simulink model "Task_2a"  (R2021b)
settings: Solver=VariableStepAuto  StartTime=0.0  StopTime=100.0  FixedStep=0.01`  RelTol=1e-3
model workspace (MAT data in the model file):
  Kd = 1
  Ki = 22
  Kp = 200
  Ts = 0.01
  b = 50
  m = 1000
  u = 500
settings Model: Creator=mluser  LastModifiedBy=mluser

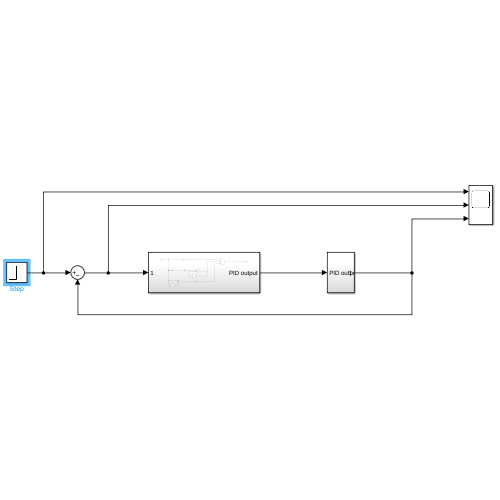
[thumbnail: Simulink's stored preview of the top-level diagram]
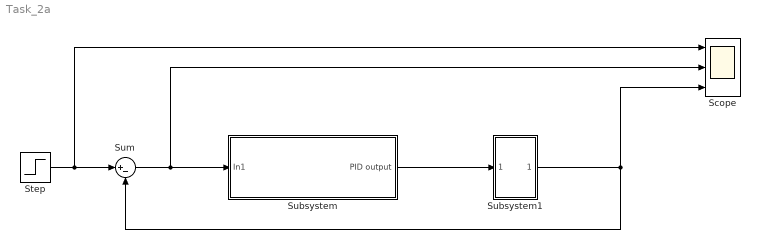
== system Task_2a ==
  Scope : Scope  NumInputPorts=3
  Step : Step  Time=0  After=u  SampleTime=0.01
  Subsystem : Subsystem
  Subsystem1 : Subsystem
  Sum : Sum  Inputs=|+-
  wires:
  Step/1 -> Sum/1, Scope/1
  Subsystem1/1(Out1) -> Sum/2, Scope/3
  Sum/1 -> Subsystem/1(In1), Scope/2
  Subsystem/1(PID output) -> Subsystem1/1(PID output)

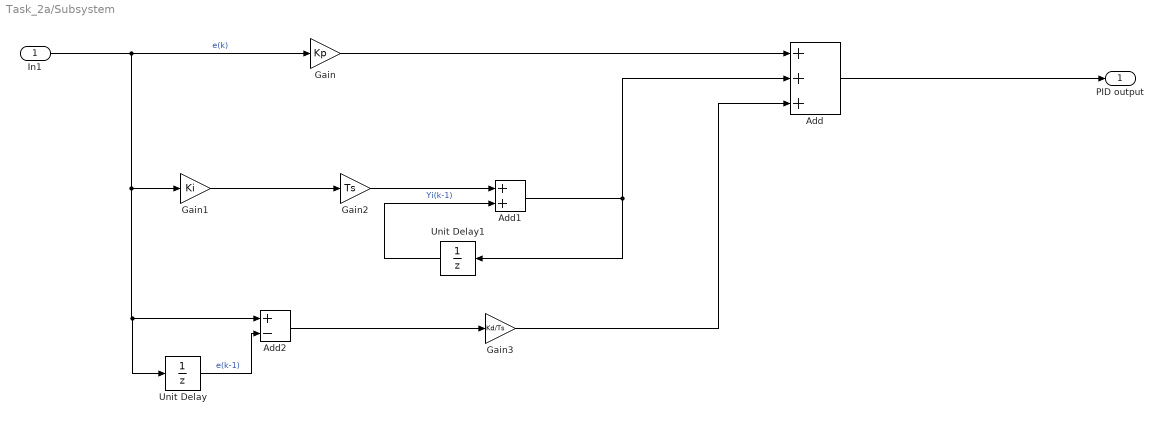
== system Task_2a/Subsystem ==
  In1 : Inport
  Add : Sum  Inputs=+++
  Add1 : Sum
  Add2 : Sum  Inputs=+-
  Gain : Gain  Gain=Kp
  Gain1 : Gain  Gain=Ki
  Gain2 : Gain  Gain=Ts
  Gain3 : Gain  Gain=Kd/Ts
  Unit Delay : UnitDelay  SampleTime=-1  HasFrameUpgradeWarning=on
  Unit Delay1 : UnitDelay  SampleTime=-1  HasFrameUpgradeWarning=on
  PID output : Outport
  wires:
  Unit Delay1/1 -> Add1/2  "Yi(k-1)"
  Gain3/1 -> Add/3
  Gain1/1 -> Gain2/1
  Unit Delay/1 -> Add2/2  "e(k-1)"
  Gain/1 -> Add/1
  In1/1 -> Unit Delay/1, Add2/1, Gain1/1, Gain/1  "e(k)"
  Add/1 -> PID output/1
  Add2/1 -> Gain3/1
  Add1/1 -> Add/2, Unit Delay1/1
  Gain2/1 -> Add1/1

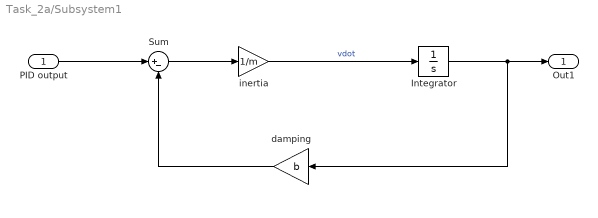
== system Task_2a/Subsystem1 ==
  PID output : Inport
  Integrator : Integrator
  Sum : Sum  Inputs=|+-
  damping : Gain  Gain=b
  inertia : Gain  Gain=1/m
  Out1 : Outport
  wires:
  damping/1 -> Sum/2
  inertia/1 -> Integrator/1  "vdot"
  Integrator/1 -> Out1/1, damping/1
  PID output/1 -> Sum/1
  Sum/1 -> inertia/1
